simulink model "sistema_completo"  (R2019a)
settings: Solver=VariableStepAuto  StartTime=0.0  StopTime=120  RelTol=1e-3
InitFcn:
  | parametros
values from neighbouring files (symbols this model uses):
  a_h_max = 0.75    [parametros.m]
  a_t_max = 0.8    [parametros.m]
  b_cx = 1.0e6    (= 1000000)    [parametros.m]
  b_cy = 1.0e7    (= 10000000)    [parametros.m]
  b_h_eq = 2 * ( b_hd + i_h^2*b_hm ) / (r_hd^2)    (= 31004.4444444)    [parametros.m]
  b_hb = 1.0e8    (= 100000000)    [parametros.m]
  b_hEb = 2.2e9    (= 2200000000)    [parametros.m]
  b_t = 90.0    (= 90)    [parametros.m]
  b_t_eq = Simulink.Parameter(b_t_eq)    [parametros.m]
  b_tb = 5.0e6    (= 5000000)    [parametros.m]
  b_td_eq = ( b_td + i_t^2*b_tm ) / (r_td^2)    (= 21607.2)    [parametros.m]
  b_tw = 3.0e3    (= 3000)    [parametros.m]
  b_wu = 150    [parametros.m]
  clearance_min = 2    [parametros.m]
  g = Simulink.Parameter(9.80665)    [parametros.m]
  H_c = Simulink.Parameter(2.59)    [parametros.m]
  i_h = 22.0    (= 22)    [parametros.m]
  i_t = 30.0    (= 30)    [parametros.m]
  K_cy = 1.8e9    (= 1800000000)    [parametros.m]
  K_d_h = 2*m_h_eq*xi_hc*w_hc + m_h_eq*p3_hc - b_h_eq    (= 221460.31746)    [parametros.m]
  K_d_t = 2*m_t_eq*xi_tc*w_tc + m_t_eq*p3_tc - b_t_eq.Value    [parametros.m]
  K_i_h = m_h_eq*p3_hc*w_hc^2    (= 25598.9338431)    [parametros.m]
  K_i_t = m_t_eq*p3_tc*w_tc^2    [parametros.m]
  k_p3_th = 3    [parametros.m]
  K_p_h = m_h_eq*w_hc^2 + 2*m_h_eq*xi_hc*w_hc*p3_hc    (= 112940.617295)    [parametros.m]
  K_p_t = m_t_eq*w_tc^2 + 2*m_t_eq*xi_tc*w_tc*p3_tc    [parametros.m]
  k_th = 1    [parametros.m]
  K_tw = 4.8e5    (= 480000)    [parametros.m]
  k_w_c_th = 0.7    [parametros.m]
  k_wu = 2.36e8    (= 236000000)    [parametros.m]
  l_h0 = Y_t0 - y_h0    [parametros.m]
  L_h0 = 110    [parametros.m]
  l_h_man_thresh = 1.0    (= 1)    [parametros.m]
  l_h_tol = 1.0    (= 1)    [parametros.m]
  M_c_max = 50000    [parametros.m]
  M_c_min = 2000    [parametros.m]
  m_h_eq = 2 * ( J_hd_hEb + i_h^2*J_hm_hb ) / (r_hd^2)    (= 65137.7777778)    [parametros.m]
  M_s = 15000    [parametros.m]
  M_t = Simulink.Parameter(30000)    [parametros.m]
  m_td_eq = ( J_td + i_t^2*J_tm_tb ) / (r_td^2)    (= 30000)    [parametros.m]
  N_slots = Simulink.Parameter(floor((x_t_max_oper.Value - x_t_min_oper.Value) / W_c.Value))    [parametros.m]
  overload = false    [parametros.m]
  P_h_nom = 956150    [parametros.m]
  r_hd = 0.75    [parametros.m]
  r_td = 0.50    (= 0.5)    [parametros.m]
  random_obstacles = false    [parametros.m]
  T_hb_max = 5.0e4    (= 50000)    [parametros.m]
  T_hEb_max = 1.1e6    (= 1100000)    [parametros.m]
  T_hm_MAX = 2.0e4    (= 20000)    [parametros.m]
  T_s1 = 20/1000    (= 0.02)    [parametros.m]
  T_s2 = 1/1000    (= 0.001)    [parametros.m]
  T_tb_max = 5.0e3    (= 5000)    [parametros.m]
  T_tm_max = 4.0e3    (= 4000)    [parametros.m]
  tau_hm = 1.0    (= 1)    [parametros.m]
  tau_tm = 1.0    (= 1)    [parametros.m]
  v_h_max = 3.0    (= 3)    [parametros.m]
  v_h_nom = 1.5    [parametros.m]
  v_t_max = 4.0    (= 4)    [parametros.m]
  W_c = Simulink.Parameter(2.44)    [parametros.m]
  w_hm_rated = 2 * (i_h / r_hd) * v_h_nom    (= 88)    [parametros.m]
  x_l0 = x_t0    [parametros.m]
  x_t0 = W_c.Value / 2    [parametros.m]
  x_t_man_thresh = 1.0    (= 1)    [parametros.m]
  x_t_max_emer = x_t_max_oper.Value + 1.0    [parametros.m]
  x_t_max_oper = Simulink.Parameter(50.0)    [parametros.m]
  x_t_min_emer = x_t_min_oper.Value - 1.0    [parametros.m]
  x_t_min_oper = Simulink.Parameter(-30.0)    [parametros.m]
  x_td0 = x_t0    [parametros.m]
  xi_c_th = 0.7    [parametros.m]
  y_c0_0 = Simulink.Parameter(y_c0_ship)    [parametros.m]
  y_c0_quay = 0    [parametros.m]
  y_c0_ship = -20    [parametros.m]
  y_h_max_emer = y_h_max_oper.Value + 1.0    [parametros.m]
  y_h_max_oper = Simulink.Parameter(40.0)    [parametros.m]
  y_h_min_emer = y_h_min_oper.Value - 1.0    [parametros.m]
  y_h_min_oper = Simulink.Parameter(-20.0)    [parametros.m]
  y_l0 = y_h0    [parametros.m]
  Y_t0 = 45.0    (= 45)    [parametros.m]
undefined symbols (not defined in the file or in its folder): DiscIntNeverNeededParam, F_hw, hoist, l_h, l_h_dot, sigbuilder_block, theta_l, theta_l_dot, TLK, translation, x_t_dot
libraries: simulink x10, vrlib x1
(part 1 of 2)
settings Model: EnablePacing=on  Creator=Facundo  LastModifiedBy=Facundo

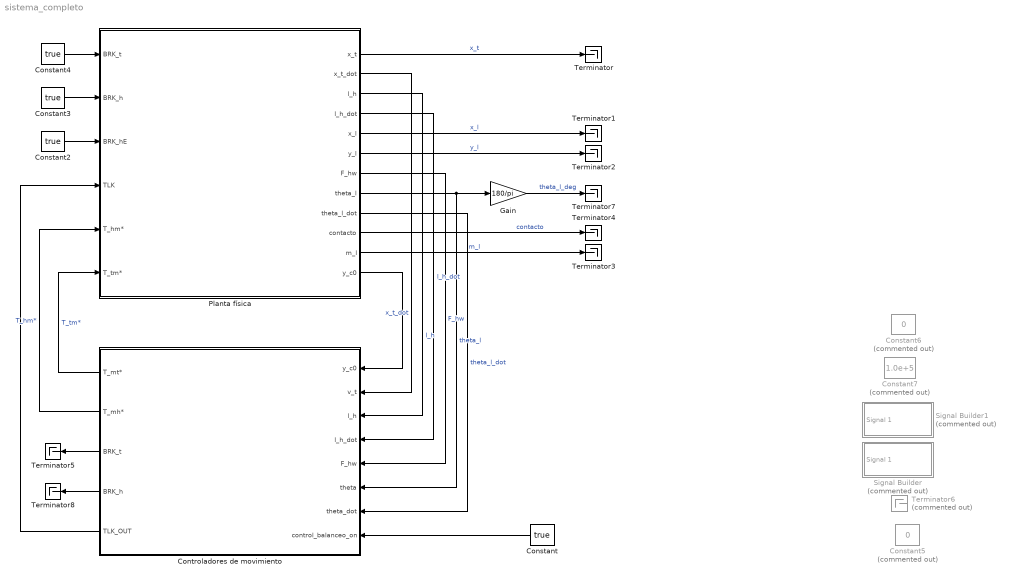
== system sistema_completo ==
  Constant{,2..4} (4 alike) : Constant  Value=true  OutDataTypeStr=boolean
  Constant5 : Constant  Commented=on  Value=0  OutDataTypeStr=boolean
  Constant6 : Constant  Commented=on  Value=0  OutDataTypeStr=double
  Constant7 : Constant  Commented=on  Value=1.0e+5  OutDataTypeStr=double
  Controladores de movimiento : Subsystem
  Gain : Gain  Gain=180/pi
  Planta física : Subsystem
  Signal Builder : Subsystem  Tag=STV Subsys  Commented=on  LoadFcn=sigbuilder_block('load');  StartFcn=sigbuilder_block('start');  StopFcn=sigbuilder_block('stop');  ClipboardFcn=sigbuilder_block('clipboard');  mask(Sigbuilder block){tuvar=[0:10]}
      mask help: Simulink:masks:SigbuilderBlock_MD
      mask init:
      | if ~strcmp(get_param(bdroot(gcbh),'SimulationStatus'),'stopped') tuvar = sigbuilder_block('maskInit'); end
      settings: CopyFcn=sigbuilder_block('copy');  DeleteFcn=sigbuilder_block('delete');  ModelCloseFcn=sigbuilder_block('modelClose');  PreSaveFcn=sigbuilder_block('preSave');  PauseFcn=sigbuilder_block('pause');  ContinueFcn=sigbuilder_block('continue');  NameChangeFcn=sigbuilder_block('namechange');  OpenFcn=sigbuilder_block('open',[5.14286 5.14286 812.571 450.429 ]);  CloseFcn=sigbuilder_block('close');
      mask Display: plot(0, 0, 100, 100,[2, 2, 32, 32, 2], [68, 8, 8, 68, 68],[32, 2], [38, 38], [32, 19, 2],[53, 60, 44], [32, 17, 17, 2],[16, 16, 31, 31]);txt = getActiveGroup(gcbh);text(2, 100, txt,'verticalAlignment', 'top');
  Signal Builder1 : Subsystem  Tag=STV Subsys  Commented=on  LoadFcn=sigbuilder_block('load');  StartFcn=sigbuilder_block('start');  StopFcn=sigbuilder_block('stop');  ClipboardFcn=sigbuilder_block('clipboard');  mask(Sigbuilder block){tuvar=[0:10]}
      mask help: Simulink:masks:SigbuilderBlock_MD
      mask init:
      | if ~strcmp(get_param(bdroot(gcbh),'SimulationStatus'),'stopped') tuvar = sigbuilder_block('maskInit'); end
      settings: CopyFcn=sigbuilder_block('copy');  DeleteFcn=sigbuilder_block('delete');  ModelCloseFcn=sigbuilder_block('modelClose');  PreSaveFcn=sigbuilder_block('preSave');  PauseFcn=sigbuilder_block('pause');  ContinueFcn=sigbuilder_block('continue');  NameChangeFcn=sigbuilder_block('namechange');  OpenFcn=sigbuilder_block('open',[-1152 -103.714 1152 564.429 ]);  CloseFcn=sigbuilder_block('close');
      mask Display: plot(0, 0, 100, 100,[2, 2, 32, 32, 2], [68, 8, 8, 68, 68],[32, 2], [38, 38], [32, 19, 2],[53, 60, 44], [32, 17, 17, 2],[16, 16, 31, 31]);txt = getActiveGroup(gcbh);text(2, 100, txt,'verticalAlignment', 'top');
  Terminator{,1..5,7..8} (8 alike) : Terminator
  Terminator6 : Terminator  Commented=on
  wires:
  Constant/1 -> Controladores de movimiento/8(control_balanceo_on)
  Controladores de movimiento/1(T_mt*) -> Planta física/6(T_tm*)  "T_tm*"
  Controladores de movimiento/2(T_mh*) -> Planta física/5(T_hm*)  "T_hm*"
  Planta física/2(x_t_dot) -> Controladores de movimiento/2(v_t)  "x_t_dot"
  Planta física/4(l_h_dot) -> Controladores de movimiento/4(l_h_dot)  "l_h_dot"
  Planta física/8(theta_l) -> Controladores de movimiento/6(theta), Gain/1  "theta_l"
  Planta física/9(theta_l_dot) -> Controladores de movimiento/7(theta_dot)  "theta_l_dot"
  Planta física/3(l_h) -> Controladores de movimiento/3(l_h)  "l_h"
  Planta física/1(x_t) -> Terminator/1  "x_t"
  Controladores de movimiento/5(TLK_OUT) -> Planta física/4(TLK)
  Constant2/1 -> Planta física/3(BRK_hE)
  Constant3/1 -> Planta física/2(BRK_h)
  Constant4/1 -> Planta física/1(BRK_t)
  Planta física/5(x_l) -> Terminator1/1  "x_l"
  Planta física/6(y_l) -> Terminator2/1  "y_l"
  Planta física/7(F_hw) -> Controladores de movimiento/5(F_hw)  "F_hw"
  Planta física/10(contacto) -> Terminator4/1  "contacto"
  Gain/1 -> Terminator7/1  "theta_l_deg"
  Planta física/11(m_l) -> Terminator3/1  "m_l"
  Controladores de movimiento/3(BRK_t) -> Terminator5/1
  Controladores de movimiento/4(BRK_h) -> Terminator8/1
  Planta física/12(y_c0) -> Controladores de movimiento/1(y_c0)

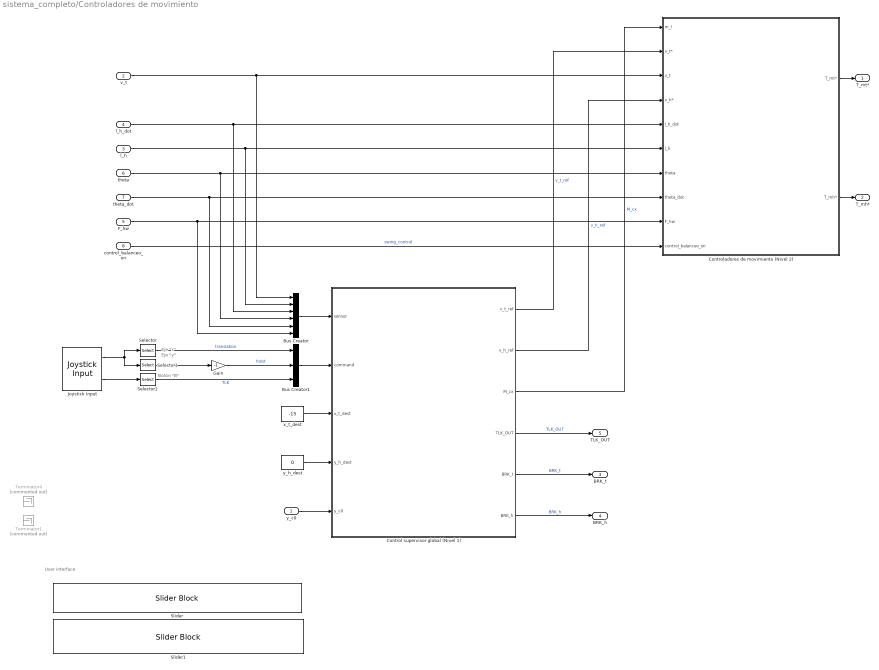
== system sistema_completo/Controladores de movimiento ==
  note: User interface
  note: Botón "B"
  note: Eje "y"
  note: Eje "x"
  y_c0 : Inport  OutDataTypeStr=boolean  LockScale=on
  v_t : Inport  Port=2
  l_h : Inport  Port=3
  l_h_dot : Inport  Port=4
  F_hw : Inport  Port=5
  theta : Inport  Port=6
  theta_dot : Inport  Port=7
  control_balanceo_on : Inport  Port=8  OutDataTypeStr=boolean  LockScale=on
  Bus Creator : BusCreator  Inputs=x_t_dot,l_h,l_h_dot,theta_l,theta_l_dot,F_hw  OutDataTypeStr=Bus: sensor_bus
  Bus Creator1 : BusCreator  Inputs=translation,hoist,TLK  OutDataTypeStr=Bus: command_bus
  Control supervisor global (Nivel 1) : Stateflow chart  BlockKeywords=__PRM__SERIALIZED__DATA__:Stateflow Chart,Stateflow Diagram  TreatAsAtomicUnit=on  SystemSampleTime=T_s1
  Controladores de movimiento (Nivel 2) : Subsystem
  Gain : Gain  Gain=-1
  Joystick Input : vrlib/Joystick Input  joyid=1  adjustports=off  forcefeed=off
      settings: SourceProductName=Simulink
  Selector : Selector  IndexOptions=Index vector (dialog)  Indices=[1]  OutputSizes=1
  Selector1 : Selector  IndexOptions=Index vector (dialog)  Indices=[2]  OutputSizes=1
  Selector2 : Selector  IndexOptions=Index vector (dialog)  Indices=[1]  OutputSizes=1
  Slider : SliderBlock  ScaleMin=-30  ScaleMax=50  TickInterval=5
  Slider1 : SliderBlock  ScaleMin=-20  ScaleMax=40  TickInterval=5
  Terminator1 : Terminator  Commented=on
  Terminator4 : Terminator  Commented=on
  x_t_dest : Constant  Value=-15  OutDataTypeStr=int32
  y_h_dest : Constant  Value=0  OutDataTypeStr=int32
  T_mt* : Outport
  T_mh* : Outport  Port=2
  BRK_t : Outport  Port=3
  BRK_h : Outport  Port=4
  TLK_OUT : Outport  Port=5  OutDataTypeStr=boolean
  wires:
  F_hw/1 -> Bus Creator/6, Controladores de movimiento (Nivel 2)/9(F_hw)
  Controladores de movimiento (Nivel 2)/2(T_mh*) -> T_mh*/1
  Controladores de movimiento (Nivel 2)/1(T_mt*) -> T_mt*/1
  theta/1 -> Bus Creator/4, Controladores de movimiento (Nivel 2)/7(theta)
  control_balanceo_on/1 -> Controladores de movimiento (Nivel 2)/10(control_balanceo_on)  "swing_control"
  theta_dot/1 -> Bus Creator/5, Controladores de movimiento (Nivel 2)/8(theta_dot)
  l_h_dot/1 -> Bus Creator/3, Controladores de movimiento (Nivel 2)/5(l_h_dot)
  v_t/1 -> Bus Creator/1, Controladores de movimiento (Nivel 2)/3(v_t)
  Bus Creator/1 -> Control supervisor global (Nivel 1)/1(sensor)
  l_h/1 -> Controladores de movimiento (Nivel 2)/6(l_h), Bus Creator/2
  Selector/1 -> Bus Creator1/1  "translation"
  Joystick Input/1 -> Selector/1, Selector1/1
  Bus Creator1/1 -> Control supervisor global (Nivel 1)/2(command)
  Control supervisor global (Nivel 1)/1(v_t_ref) -> Controladores de movimiento (Nivel 2)/2(v_t*)  "v_t_ref"
  Control supervisor global (Nivel 1)/2(v_h_ref) -> Controladores de movimiento (Nivel 2)/4(v_h*)  "v_h_ref"
  Control supervisor global (Nivel 1)/5(BRK_t) -> BRK_t/1  "BRK_t"
  Control supervisor global (Nivel 1)/6(BRK_h) -> BRK_h/1  "BRK_h"
  Control supervisor global (Nivel 1)/4(TLK_OUT) -> TLK_OUT/1  "TLK_OUT"
  Control supervisor global (Nivel 1)/3(M_cx) -> Controladores de movimiento (Nivel 2)/1(m_l)  "M_cx"
  Joystick Input/2 -> Selector2/1
  Selector1/1 -> Gain/1
  Selector2/1 -> Bus Creator1/3  "TLK"
  Gain/1 -> Bus Creator1/2  "hoist"
  x_t_dest/1 -> Control supervisor global (Nivel 1)/3(x_t_dest)
  y_h_dest/1 -> Control supervisor global (Nivel 1)/4(y_h_dest)
  y_c0/1 -> Control supervisor global (Nivel 1)/5(y_c0)

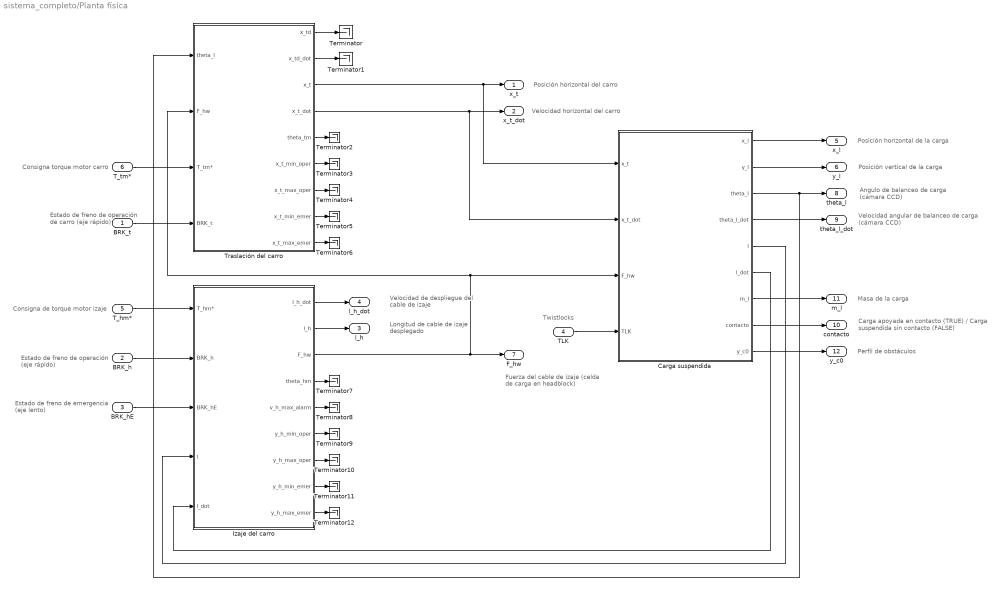
== system sistema_completo/Planta física ==
  note: Consigna de torque motor izaje
  note: Posición horizontal del carro
  note: Velocidad de despliegue
      | del cable de izaje
  note: Longitud de cable
      | de izaje desplegado
  note: Posición horizontal de la carga
  note: Fuerza del cable de izaje
      | (celda de carga en headblock)
  note: Estado de freno de emergencia
      | (eje lento)
  note: Twistlocks
  note: Estado de freno de operación
      | (eje rápido)
  note: Ángulo de balanceo de carga
      | (cámara CCD)
  note: Consigna torque motor carro
  note: Estado de freno de
      | operación de carro
      | (eje rápido)
  note: Posición vertical de la carga
  note: Velocidad horizontal del carro
  note: Velocidad angular de balanceo de carga
      | (cámara CCD)
  note: Masa de la carga
  note: Carga apoyada en contacto (TRUE) /
      | Carga suspendida sin contacto (FALSE)
  note: Perfil de obstáculos
  BRK_t : Inport
  BRK_h : Inport  Port=2
  BRK_hE : Inport  Port=3
  TLK : Inport  Port=4  OutDataTypeStr=boolean  PortDimensions=1  SampleTime=0
  T_hm* : Inport  Port=5
  T_tm* : Inport  Port=6
  Carga suspendida : Subsystem
  Izaje del carro : Subsystem
  Terminator{,1..12} (13 alike) : Terminator
  Traslación del carro : Subsystem
  x_t : Outport
  x_t_dot : Outport  Port=2
  l_h : Outport  Port=3
  l_h_dot : Outport  Port=4
  x_l : Outport  Port=5
  y_l : Outport  Port=6
  F_hw : Outport  Port=7
  theta_l : Outport  Port=8
  theta_l_dot : Outport  Port=9
  contacto : Outport  Port=10
  m_l : Outport  Port=11
  y_c0 : Outport  Port=12
  wires:
  BRK_hE/1 -> Izaje del carro/3(BRK_hE)
  BRK_h/1 -> Izaje del carro/2(BRK_h)
  Traslación del carro/3(x_t) -> Carga suspendida/1(x_t), x_t/1
  BRK_t/1 -> Traslación del carro/4(BRK_t)
  Traslación del carro/1(x_td) -> Terminator/1
  Izaje del carro/1(l_h_dot) -> l_h_dot/1
  Izaje del carro/3(F_hw) -> F_hw/1, Traslación del carro/2(F_hw), Carga suspendida/3(F_hw)
  Carga suspendida/6(l_dot) -> Izaje del carro/5(l_dot)
  Carga suspendida/5(l) -> Izaje del carro/4(l)
  TLK/1 -> Carga suspendida/4(TLK)
  Carga suspendida/3(theta_l) -> Traslación del carro/1(theta_l), theta_l/1
  T_hm*/1 -> Izaje del carro/1(T_hm*)
  Carga suspendida/1(x_l) -> x_l/1
  Izaje del carro/2(l_h) -> l_h/1
  Carga suspendida/2(y_l) -> y_l/1
  Traslación del carro/4(x_t_dot) -> Carga suspendida/2(x_t_dot), x_t_dot/1
  Traslación del carro/2(x_td_dot) -> Terminator1/1
  T_tm*/1 -> Traslación del carro/3(T_tm*)
  Traslación del carro/5(theta_tm) -> Terminator2/1
  Traslación del carro/6(x_t_min_oper) -> Terminator3/1
  Traslación del carro/7(x_t_max_oper) -> Terminator4/1
  Traslación del carro/8(x_t_min_emer) -> Terminator5/1
  Traslación del carro/9(x_t_max_emer) -> Terminator6/1
  Izaje del carro/4(theta_hm) -> Terminator7/1
  Izaje del carro/5(v_h_max_alarm) -> Terminator8/1
  Izaje del carro/6(y_h_min_oper) -> Terminator9/1
  Izaje del carro/7(y_h_max_oper) -> Terminator10/1
  Izaje del carro/8(y_h_min_emer) -> Terminator11/1
  Izaje del carro/9(y_h_max_emer) -> Terminator12/1
  Carga suspendida/4(theta_l_dot) -> theta_l_dot/1
  Carga suspendida/8(contacto) -> contacto/1
  Carga suspendida/7(m_l) -> m_l/1
  Carga suspendida/9(y_c0) -> y_c0/1

== system sistema_completo/Signal Builder ==
  Demux : Demux  Tag=STV Demux  Outputs=1
  FromWs : FromWorkspace  Tag=STV FromWs  VariableName=tuvar  SampleTime=0
      SigBuilderData=|
      | common.afterFinalStr = 'Extrapolate'
      | common.sampleTime = 0
      | dataSet.timeRange = [0 60]
      | dataSet.name = 'Group 1'
      | sbobj.Groups.Name = 'Group 1'
      | sbobj.Groups.Signals.Name = 'Signal 1'
      | sbobj.Groups.Signals.XData = [0 5 15 35 45 60]
      | sbobj.Groups.Signals.YData = [0 0 1 1 0 0]
      | sbobj.Groups.TimeRange = [0 60]
  Signal 1 : Outport  Tag=STV Outport
  wires:
  FromWs/1 -> Demux/1
  Demux/1 -> Signal 1/1

== system sistema_completo/Signal Builder1 ==
  Demux : Demux  Tag=STV Demux  Outputs=1
  FromWs : FromWorkspace  Tag=STV FromWs  VariableName=tuvar  SampleTime=0
      SigBuilderData=|
      | common.afterFinalStr = 'Extrapolate'
      | common.sampleTime = 0
      | dataSet.timeRange = [0 60]
      | dataSet.name = 'Group 1'
      | sbobj.Groups.Name = 'Group 1'
      | sbobj.Groups.Signals.Name = 'Signal 1'
      | sbobj.Groups.Signals.XData = [0 10 20 30 40 60]
      | sbobj.Groups.Signals.YData = [0 0 1 1 0 0]
      | sbobj.Groups.TimeRange = [0 60]
  Signal 1 : Outport  Tag=STV Outport
  wires:
  Demux/1 -> Signal 1/1
  FromWs/1 -> Demux/1

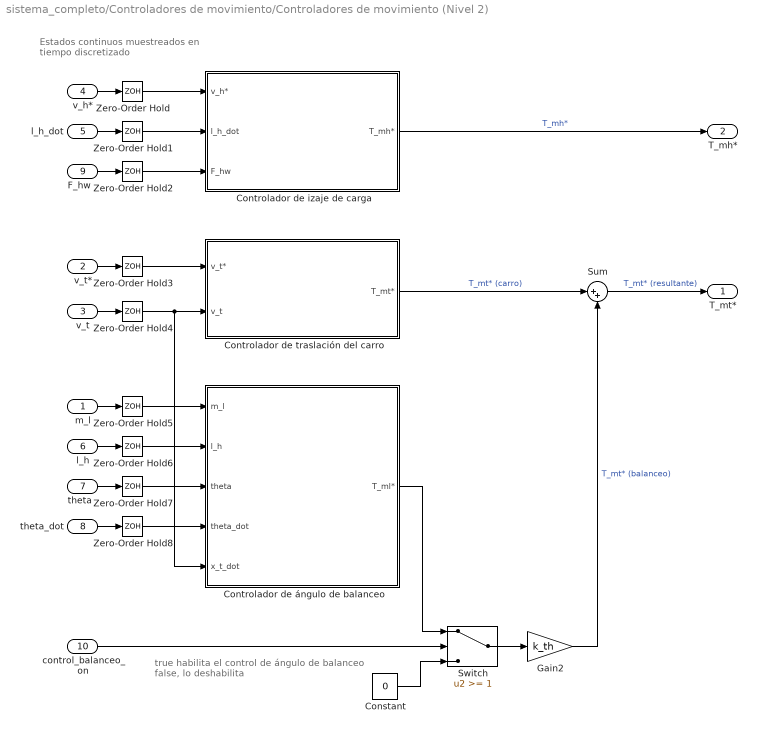
== system sistema_completo/Controladores de movimiento/Controladores de movimiento (Nivel 2) ==
  note: true habilita el control de ángulo de balanceo
      | false, lo deshabilita
  note: Estados continuos muestreados
      | en tiempo discretizado
  m_l : Inport
  v_t* : Inport  Port=2
  v_t : Inport  Port=3
  v_h* : Inport  Port=4
  l_h_dot : Inport  Port=5
  l_h : Inport  Port=6
  theta : Inport  Port=7
  theta_dot : Inport  Port=8
  F_hw : Inport  Port=9
  control_balanceo_on : Inport  Port=10  OutDataTypeStr=boolean  LockScale=on
  Constant : Constant  Value=0
  Controlador de izaje de carga : Subsystem
  Controlador de traslación del carro : Subsystem
  Controlador de ángulo de balanceo : Subsystem
  Gain2 : Gain  Gain=k_th
  Sum : Sum  Inputs=|++
  Switch : Switch  Threshold=1
  Zero-Order Hold{,1..8} (9 alike) : ZeroOrderHold  SampleTime=T_s2
  T_mt* : Outport
  T_mh* : Outport  Port=2
  wires:
  Zero-Order Hold8/1 -> Controlador de ángulo de balanceo/4(theta_dot)
  l_h_dot/1 -> Zero-Order Hold1/1
  Zero-Order Hold5/1 -> Controlador de ángulo de balanceo/1(m_l)
  Zero-Order Hold4/1 -> Controlador de ángulo de balanceo/5(x_t_dot), Controlador de traslación del carro/2(v_t)
  v_t*/1 -> Zero-Order Hold3/1
  theta/1 -> Zero-Order Hold7/1
  Constant/1 -> Switch/3
  Zero-Order Hold3/1 -> Controlador de traslación del carro/1(v_t*)
  v_h*/1 -> Zero-Order Hold/1
  v_t/1 -> Zero-Order Hold4/1
  Zero-Order Hold6/1 -> Controlador de ángulo de balanceo/2(l_h)
  Zero-Order Hold7/1 -> Controlador de ángulo de balanceo/3(theta)
  theta_dot/1 -> Zero-Order Hold8/1
  Sum/1 -> T_mt*/1  "T_mt* (resultante)"
  Zero-Order Hold1/1 -> Controlador de izaje de carga/2(l_h_dot)
  Controlador de izaje de carga/1(T_mh*) -> T_mh*/1  "T_mh*"
  Controlador de traslación del carro/1(T_mt*) -> Sum/1  "T_mt* (carro)"
  m_l/1 -> Zero-Order Hold5/1
  Switch/1 -> Gain2/1
  l_h/1 -> Zero-Order Hold6/1
  Controlador de ángulo de balanceo/1(T_ml*) -> Switch/1
  F_hw/1 -> Zero-Order Hold2/1
  Gain2/1 -> Sum/2  "T_mt* (balanceo)"
  Zero-Order Hold/1 -> Controlador de izaje de carga/1(v_h*)
  Zero-Order Hold2/1 -> Controlador de izaje de carga/3(F_hw)
  control_balanceo_on/1 -> Switch/2

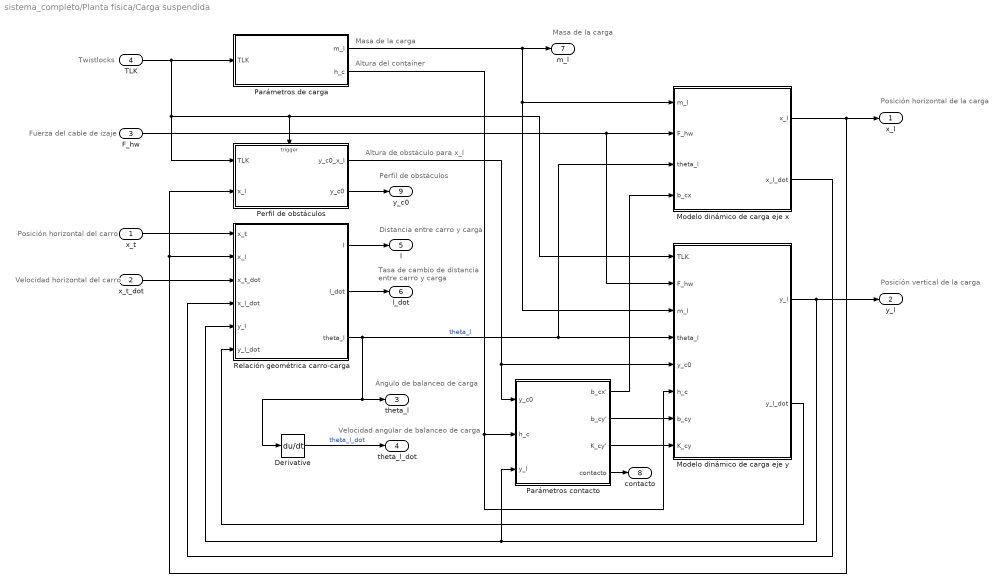
== system sistema_completo/Planta física/Carga suspendida ==
  note: Altura de obstáculo para x_l
  note: Masa de la carga
  note: Twistlocks
  note: Altura del container
  note: Posición horizontal del carro
  note: Posición vertical de la carga
  note: Velocidad horizontal del carro
  note: Distancia entre carro y carga
  note: Fuerza del cable de izaje
  note: Ángulo de balanceo de carga
  note: Tasa de cambio de distancia
      | entre carro y carga
  note: Masa de la carga
  note: Posición horizontal de la carga
  note: Velocidad angular de balanceo de carga
  note: Perfil de obstáculos
  x_t : Inport  OutDataTypeStr=double  PortDimensions=1  SampleTime=0
  x_t_dot : Inport  Port=2  OutDataTypeStr=double  PortDimensions=1  SampleTime=0
  F_hw : Inport  Port=3  OutDataTypeStr=double  PortDimensions=1  SampleTime=0
  TLK : Inport  Port=4  OutDataTypeStr=boolean  PortDimensions=1  SampleTime=0
  Derivative : Derivative
  Modelo dinámico de carga eje x : Subsystem
  Modelo dinámico de carga eje y : Subsystem
  Parámetros contacto : Subsystem
  Parámetros de carga : Subsystem
  Perfil de obstáculos : Subsystem
  Relación geométrica carro-carga : Subsystem
  x_l : Outport  OutDataTypeStr=double  PortDimensions=1  SampleTime=0
  y_l : Outport  Port=2  OutDataTypeStr=double  PortDimensions=1  SampleTime=0
  theta_l : Outport  Port=3  OutDataTypeStr=double  PortDimensions=1  SampleTime=0
  theta_l_dot : Outport  Port=4  OutDataTypeStr=double  PortDimensions=1  SampleTime=0
  l : Outport  Port=5  OutDataTypeStr=double  PortDimensions=1  SampleTime=0
  l_dot : Outport  Port=6  OutDataTypeStr=double  PortDimensions=1  SampleTime=0
  m_l : Outport  Port=7  OutDataTypeStr=double  PortDimensions=1  SampleTime=0
  contacto : Outport  Port=8  OutDataTypeStr=boolean  PortDimensions=1  SampleTime=0
  y_c0 : Outport  Port=9  OutDataTypeStr=double  PortDimensions=1  SampleTime=0
  wires:
  Parámetros de carga/1(m_l) -> Modelo dinámico de carga eje y/3(m_l), Modelo dinámico de carga eje x/1(m_l), m_l/1
  F_hw/1 -> Modelo dinámico de carga eje y/2(F_hw), Modelo dinámico de carga eje x/2(F_hw)
  Relación geométrica carro-carga/2(l_dot) -> l_dot/1
  x_t_dot/1 -> Relación geométrica carro-carga/3(x_t_dot)
  Modelo dinámico de carga eje y/1(y_l) -> Parámetros contacto/3(y_l), Relación geométrica carro-carga/5(y_l), y_l/1
  Modelo dinámico de carga eje x/2(x_l_dot) -> Relación geométrica carro-carga/4(x_l_dot)
  Modelo dinámico de carga eje y/2(y_l_dot) -> Relación geométrica carro-carga/6(y_l_dot)
  x_t/1 -> Relación geométrica carro-carga/1(x_t)
  Modelo dinámico de carga eje x/1(x_l) -> x_l/1, Perfil de obstáculos/2(x_l), Relación geométrica carro-carga/2(x_l)
  Relación geométrica carro-carga/3(theta_l) -> Derivative/1, theta_l/1, Modelo dinámico de carga eje x/3(theta_l), Modelo dinámico de carga eje y/4(theta_l)  "theta_l"
  Parámetros contacto/1(b_cx') -> Modelo dinámico de carga eje x/4(b_cx)
  Parámetros contacto/2(b_cy') -> Modelo dinámico de carga eje y/7(b_cy)
  Parámetros contacto/3(K_cy') -> Modelo dinámico de carga eje y/8(K_cy)
  Relación geométrica carro-carga/1(l) -> l/1
  Parámetros contacto/4(contacto) -> contacto/1
  Parámetros de carga/2(h_c) -> Parámetros contacto/2(h_c), Modelo dinámico de carga eje y/6(h_c)
  Perfil de obstáculos/1(y_c0_x_l) -> Parámetros contacto/1(y_c0), Modelo dinámico de carga eje y/5(y_c0)
  TLK/1 -> Perfil de obstáculos/1(TLK), Perfil de obstáculos/Trigger, Modelo dinámico de carga eje y/1(TLK), Parámetros de carga/1(TLK)
  Derivative/1 -> theta_l_dot/1  "theta_l_dot"
  Perfil de obstáculos/2(y_c0) -> y_c0/1

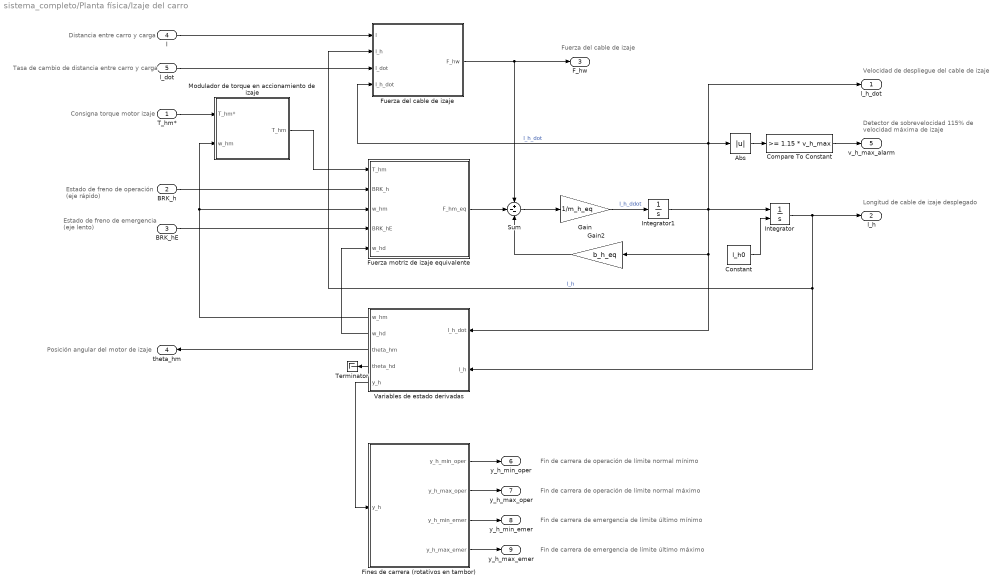
== system sistema_completo/Planta física/Izaje del carro ==
  note: Detector de sobrevelocidad
      | 115% de velocidad máxima de izaje
  note: Posición angular del motor de izaje
  note: Longitud de cable de izaje desplegado
  note: Velocidad de despliegue del cable de izaje
  note: Consigna torque motor izaje
  note: Estado de freno de emergencia
      | (eje lento)
  note: Tasa de cambio de distancia entre carro y carga
  note: Estado de freno de operación
      | (eje rápido)
  note: Distancia entre carro y carga
  note: Fuerza del cable de izaje
  note: Fin de carrera de operación de límite normal mínimo
  note: Fin de carrera de emergencia de límite último máximo
  note: Fin de carrera de emergencia de límite último mínimo
  note: Fin de carrera de operación de límite normal máximo
  T_hm* : Inport
  BRK_h : Inport  Port=2
  BRK_hE : Inport  Port=3
  l : Inport  Port=4
  l_dot : Inport  Port=5
  Abs : Abs
  Compare To Constant : simulink/Logic and Bit Operations/Compare To Constant  relop=>=  const=1.15 * v_h_max  OutDataTypeStr=boolean
  Constant : Constant  Value=l_h0
  Fines de carrera (rotativos en tambor) : Subsystem
  Fuerza del cable de izaje : Subsystem
  Fuerza motriz de izaje equivalente : Subsystem
  Gain : Gain  Gain=1/m_h_eq
  Gain2 : Gain  Gain=b_h_eq
  Integrator : Integrator  InitialConditionSource=external
  Integrator1 : Integrator
  Modulador de torque en accionamiento de izaje : Subsystem
  Sum : Sum  Inputs=+--
  Terminator : Terminator
  Variables de estado derivadas : Subsystem
  l_h_dot : Outport
  l_h : Outport  Port=2
  F_hw : Outport  Port=3
  theta_hm : Outport  Port=4
  v_h_max_alarm : Outport  Port=5
  y_h_min_oper : Outport  Port=6  OutDataTypeStr=boolean  PortDimensions=1  SampleTime=0
  y_h_max_oper : Outport  Port=7  OutDataTypeStr=boolean  PortDimensions=1  SampleTime=0
  y_h_min_emer : Outport  Port=8  OutDataTypeStr=boolean  PortDimensions=1  SampleTime=0
  y_h_max_emer : Outport  Port=9  OutDataTypeStr=boolean  PortDimensions=1  SampleTime=0
  wires:
  Integrator/1 -> l_h/1, Variables de estado derivadas/2(l_h), Fuerza del cable de izaje/2(l_h)  "l_h"
  Integrator1/1 -> l_h_dot/1, Fuerza del cable de izaje/4(l_h_dot), Abs/1, Variables de estado derivadas/1(l_h_dot), Gain2/1, Integrator/1  "l_h_dot"
  l/1 -> Fuerza del cable de izaje/1(l)
  l_dot/1 -> Fuerza del cable de izaje/3(l_dot)
  Fuerza del cable de izaje/1(F_hw) -> F_hw/1, Sum/1
  Gain2/1 -> Sum/3
  Fuerza motriz de izaje equivalente/1(F_hm_eq) -> Sum/2
  Variables de estado derivadas/1(w_hm) -> Fuerza motriz de izaje equivalente/3(w_hm), Modulador de torque en accionamiento de izaje/2(w_hm)
  Sum/1 -> Gain/1
  Variables de estado derivadas/2(w_hd) -> Fuerza motriz de izaje equivalente/5(w_hd)
  BRK_h/1 -> Fuerza motriz de izaje equivalente/2(BRK_h)
  BRK_hE/1 -> Fuerza motriz de izaje equivalente/4(BRK_hE)
  Gain/1 -> Integrator1/1  "l_h_ddot"
  Constant/1 -> Integrator/2
  Variables de estado derivadas/3(theta_hm) -> theta_hm/1
  Abs/1 -> Compare To Constant/1
  Compare To Constant/1 -> v_h_max_alarm/1
  Fines de carrera (rotativos en tambor)/1(y_h_min_oper) -> y_h_min_oper/1
  Fines de carrera (rotativos en tambor)/4(y_h_max_emer) -> y_h_max_emer/1
  Fines de carrera (rotativos en tambor)/3(y_h_min_emer) -> y_h_min_emer/1
  Fines de carrera (rotativos en tambor)/2(y_h_max_oper) -> y_h_max_oper/1
  Variables de estado derivadas/5(y_h) -> Fines de carrera (rotativos en tambor)/1(y_h)
  Variables de estado derivadas/4(theta_hd) -> Terminator/1
  Modulador de torque en accionamiento de izaje/1(T_hm) -> Fuerza motriz de izaje equivalente/1(T_hm)
  T_hm*/1 -> Modulador de torque en accionamiento de izaje/1(T_hm*)

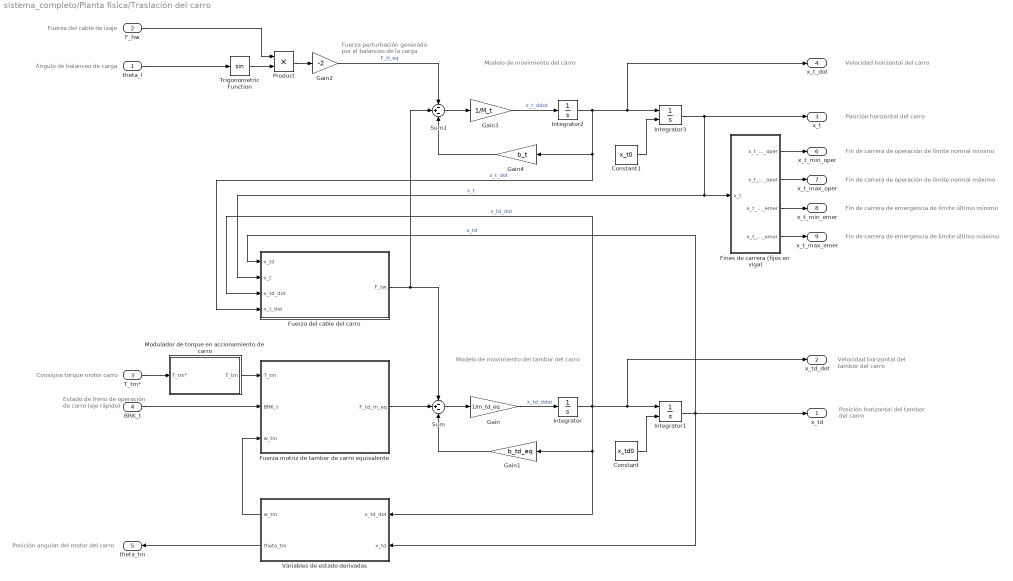
== system sistema_completo/Planta física/Traslación del carro ==
  note: Posición angular del motor del carro
  note: Velocidad horizontal
      | del tambor del carro
  note: Modelo de movimiento del tambor del carro
  note: Modelo de movimiento del carro
  note: Velocidad horizontal del carro
  note: Estado de freno de
      | operación de carro
      | (eje rápido)
  note: Fuerza del cable de izaje
  note: Fuerza perturbación generada
      | por el balanceo de la carga
  note: Posición horizontal del carro
  note: Consigna torque motor carro
  note: Ángulo de balanceo de carga
  note: Posición horizontal
      | del tambor del carro
  note: Fin de carrera de operación de límite normal mínimo
  note: Fin de carrera de operación de límite normal máximo
  note: Fin de carrera de emergencia de límite último mínimo
  note: Fin de carrera de emergencia de límite último máximo
  theta_l : Inport  OutDataTypeStr=double  PortDimensions=1  SampleTime=0
  F_hw : Inport  Port=2  OutDataTypeStr=double  PortDimensions=1  SampleTime=0
  T_tm* : Inport  Port=3
  BRK_t : Inport  Port=4
  Constant : Constant  Value=x_td0
  Constant1 : Constant  Value=x_t0
  Fines de carrera (fijos en viga) : Subsystem
  Fuerza del cable del carro : Subsystem
  Fuerza motriz de tambor de carro equivalente : Subsystem
  Gain : Gain  Gain=1/m_td_eq
  Gain1 : Gain  Gain=b_td_eq
  Gain2 : Gain  Gain=-2
  Gain3 : Gain  Gain=1/M_t
  Gain4 : Gain  Gain=b_t
  Integrator : Integrator
  Integrator1 : Integrator  InitialConditionSource=external
  Integrator2 : Integrator
  Integrator3 : Integrator  InitialConditionSource=external
  Modulador de torque en accionamiento de carro : Subsystem
  Product : Product
  Sum : Sum  Inputs=-+-
  Sum1 : Sum  Inputs=-+-
  Trigonometric Function : Trigonometry
  Variables de estado derivadas : Subsystem
  x_td : Outport  OutDataTypeStr=double  PortDimensions=1  SampleTime=0
  x_td_dot : Outport  Port=2  OutDataTypeStr=double  PortDimensions=1  SampleTime=0
  x_t : Outport  Port=3  OutDataTypeStr=double  PortDimensions=1  SampleTime=0
  x_t_dot : Outport  Port=4  OutDataTypeStr=double  PortDimensions=1  SampleTime=0
  theta_tm : Outport  Port=5  OutDataTypeStr=double  PortDimensions=1  SampleTime=0
  x_t_min_oper : Outport  Port=6  OutDataTypeStr=boolean  PortDimensions=1  SampleTime=0
  x_t_max_oper : Outport  Port=7  OutDataTypeStr=boolean  PortDimensions=1  SampleTime=0
  x_t_min_emer : Outport  Port=8  OutDataTypeStr=boolean  PortDimensions=1  SampleTime=0
  x_t_max_emer : Outport  Port=9  OutDataTypeStr=boolean  PortDimensions=1  SampleTime=0
  wires:
  Integrator1/1 -> Variables de estado derivadas/2(x_td), Fuerza del cable del carro/1(x_td), x_td/1  "x_td"
  Gain3/1 -> Integrator2/1  "x_t_ddot"
  Fuerza del cable del carro/1(F_tw) -> Sum1/2, Sum/1
  Sum/1 -> Gain/1
  Integrator/1 -> Fuerza del cable del carro/3(x_td_dot), Variables de estado derivadas/1(x_td_dot), Gain1/1, x_td_dot/1, Integrator1/1  "x_td_dot"
  F_hw/1 -> Product/1
  Fuerza motriz de tambor de carro equivalente/1(F_td_m_eq) -> Sum/2
  Constant/1 -> Integrator1/2
  Gain1/1 -> Sum/3
  Integrator2/1 -> Fuerza del cable del carro/4(x_t_dot), Gain4/1, x_t_dot/1, Integrator3/1  "x_t_dot"
  Sum1/1 -> Gain3/1
  theta_l/1 -> Trigonometric Function/1
  Gain4/1 -> Sum1/3
  Integrator3/1 -> x_t/1, Fuerza del cable del carro/2(x_t), Fines de carrera (fijos en viga)/1(x_t)  "x_t"
  Gain2/1 -> Sum1/1  "F_tl_eq"
  T_tm*/1 -> Modulador de torque en accionamiento de carro/1(T_tm*)
  BRK_t/1 -> Fuerza motriz de tambor de carro equivalente/2(BRK_t)
  Variables de estado derivadas/1(w_tm) -> Fuerza motriz de tambor de carro equivalente/3(w_tm)
  Constant1/1 -> Integrator3/2
  Trigonometric Function/1 -> Product/2
  Product/1 -> Gain2/1
  Gain/1 -> Integrator/1  "x_td_ddot"
  Variables de estado derivadas/2(theta_tm) -> theta_tm/1
  Fines de carrera (fijos en viga)/1(x_t_min_oper) -> x_t_min_oper/1
  Fines de carrera (fijos en viga)/2(x_t_max_oper) -> x_t_max_oper/1
  Fines de carrera (fijos en viga)/3(x_t_min_emer) -> x_t_min_emer/1
  Fines de carrera (fijos en viga)/4(x_t_max_emer) -> x_t_max_emer/1
  Modulador de torque en accionamiento de carro/1(T_tm) -> Fuerza motriz de tambor de carro equivalente/1(T_tm)

== system sistema_completo/Controladores de movimiento/Controladores de movimiento (Nivel 2)/Controlador de izaje de carga ==
  v_h* : Inport
  l_h_dot : Inport  Port=2
  F_hw : Inport  Port=3
  Discrete-Time Integrator : DiscreteIntegrator  SampleTime=T_s2  ICPrevOutput=DiscIntNeverNeededParam  ICPrevScaledInput=DiscIntNeverNeededParam
  Discrete-Time Integrator1 : DiscreteIntegrator  SampleTime=T_s2  ICPrevOutput=DiscIntNeverNeededParam  ICPrevScaledInput=DiscIntNeverNeededParam
  Gain : Gain  Gain=K_d_h
  Gain1 : Gain  Gain=-1
  Gain2 : Gain  Gain=K_p_h
  Gain3 : Gain  Gain=K_i_h
  Gain5 : Gain  Gain=r_hd/i_h
  Sum : Sum  Inputs=+++
  Sum1 : Sum  Inputs=|+-
  Sum2 : Sum  Inputs=|-+
  T_mh* : Outport
  wires:
  Discrete-Time Integrator1/1 -> Gain3/1
  Gain/1 -> Sum/3  "acción D"
  v_h*/1 -> Gain1/1  "v_h*"
  Discrete-Time Integrator/1 -> Gain2/1, Discrete-Time Integrator1/1
  Gain3/1 -> Sum/1  "acción I"
  Gain2/1 -> Sum/2  "acción P"
  Sum/1 -> Sum2/1  "F_h_eq_total*"
  Sum1/1 -> Discrete-Time Integrator/1, Gain/1  "e_l_h"
  Gain1/1 -> Sum1/1  "l_h_dot*"
  l_h_dot/1 -> Sum1/2  "l_h_dot"
  Gain5/1 -> T_mh*/1  "T_mh*"
  F_hw/1 -> Sum2/2  "F_hw"
  Sum2/1 -> Gain5/1

== system sistema_completo/Controladores de movimiento/Controladores de movimiento (Nivel 2)/Controlador de traslación del carro ==
  v_t* : Inport
  v_t : Inport  Port=2
  Discrete-Time Integrator : DiscreteIntegrator  SampleTime=T_s2  ICPrevOutput=DiscIntNeverNeededParam  ICPrevScaledInput=DiscIntNeverNeededParam
  Discrete-Time Integrator1 : DiscreteIntegrator  SampleTime=T_s2  ICPrevOutput=DiscIntNeverNeededParam  ICPrevScaledInput=DiscIntNeverNeededParam
  Gain : Gain  Gain=K_d_t
  Gain1 : Gain  Gain=r_td/i_t
  Gain2 : Gain  Gain=K_p_t
  Gain3 : Gain  Gain=K_i_t
  Sum : Sum  Inputs=+++
  Sum1 : Sum  Inputs=|+-
  T_mt* : Outport
  wires:
  v_t/1 -> Sum1/2
  Discrete-Time Integrator/1 -> Discrete-Time Integrator1/1, Gain2/1
  Gain2/1 -> Sum/2  "acción P"
  Gain3/1 -> Sum/1  "acción I"
  Sum1/1 -> Discrete-Time Integrator/1, Gain/1  "e_v_t"
  v_t*/1 -> Sum1/1
  Discrete-Time Integrator1/1 -> Gain3/1
  Gain/1 -> Sum/3  "acción D"
  Sum/1 -> Gain1/1  "F_t_eq*"
  Gain1/1 -> T_mt*/1  "T_mt*"

== system sistema_completo/Controladores de movimiento/Controladores de movimiento (Nivel 2)/Controlador de ángulo de balanceo ==
  note: Entrada virtual
      | al subsistema
  note: Nota:
      | e_theta = theta* - theta
      | theta* = 0 (consigna)
      |
      | Entonces
      | e_theta = - theta
      | e_theta_dot = - theta_dot
  note: Variable de ajuste
  note: Salida del
      | subsistema
  note: Entrada real
      | al subsistema
  m_l : Inport
  l_h : Inport  Port=2
  theta : Inport  Port=3
  theta_dot : Inport  Port=4
  x_t_dot : Inport  Port=5
  Des-linearización por retroalimentación : Subsystem
  Discrete-Time Integrator : DiscreteIntegrator  SampleTime=T_s2  ICPrevOutput=DiscIntNeverNeededParam  ICPrevScaledInput=DiscIntNeverNeededParam
  Gain : Gain  Gain=-1
  Gain1 : Gain  Gain=-1
  Gain2 : Gain  Gain=r_td/i_t
  Ganancias programadas : Subsystem
  Product : Product
  Product1 : Product
  Product2 : Product
  Sum : Sum  Inputs=+++
  T_ml* : Outport
  wires:
  Product1/1 -> Sum/2  "acción P"
  Product/1 -> Sum/1  "acción I"
  Discrete-Time Integrator/1 -> Product/2
  Product2/1 -> Sum/3  "acción D"
  Ganancias programadas/1(K_p_th) -> Product/1
  Ganancias programadas/2(K_i_th) -> Product1/1
  Ganancias programadas/3(K_d_th) -> Product2/1
  l_h/1 -> Des-linearización por retroalimentación/6(l_h), Ganancias programadas/1(l_h)
  Gain1/1 -> Product2/2  "e_theta_dot"
  theta/1 -> Gain/1
  theta_dot/1 -> Des-linearización por retroalimentación/4(theta_dot), Gain1/1
  Sum/1 -> Des-linearización por retroalimentación/2(v)  "v(t)"
  x_t_dot/1 -> Des-linearización por retroalimentación/5(x_t_dot)
  Des-linearización por retroalimentación/1(F_t_eq) -> Gain2/1
  Gain2/1 -> T_ml*/1
  m_l/1 -> Des-linearización por retroalimentación/1(m_l)
  Gain/1 -> Discrete-Time Integrator/1, Product1/2, Des-linearización por retroalimentación/3(theta)  "e_theta"

== system sistema_completo/Planta física/Carga suspendida/Modelo dinámico de carga eje x ==
  note: Componente horizontal de
      | fuerza del cable de izaje
  note: Posición horizontal de la carga
  note: Velocidad horizontal de la carga
  note: Fuerza del cable de izaje
  note: Masa de la carga
  note: Fricción por contacto
      | horizontal (arrastre)
  note: Ángulo de balanceo de carga
  m_l : Inport  OutDataTypeStr=double  PortDimensions=1  SampleTime=0
  F_hw : Inport  Port=2  OutDataTypeStr=double  PortDimensions=1  SampleTime=0
  theta_l : Inport  Port=3  OutDataTypeStr=double  PortDimensions=1  SampleTime=0
  b_cx : Inport  Port=4  OutDataTypeStr=double  PortDimensions=1  SampleTime=0
  Constant : Constant  Value=x_l0
  Divide : Product  Inputs=*/
  Gain2 : Gain  Gain=-2
  Integrator : Integrator
  Integrator1 : Integrator  InitialConditionSource=external
  Product : Product
  Product1 : Product
  Sum : Sum  Inputs=|+-
  Trigonometric Function : Trigonometry
  x_l : Outport  OutDataTypeStr=double  PortDimensions=1  SampleTime=0
  x_l_dot : Outport  Port=2  OutDataTypeStr=double  PortDimensions=1  SampleTime=0
  wires:
  F_hw/1 -> Product/1
  Product1/1 -> Sum/2
  theta_l/1 -> Trigonometric Function/1
  b_cx/1 -> Product1/2
  Sum/1 -> Divide/1
  Integrator/1 -> x_l_dot/1, Integrator1/1, Product1/1  "x_l_dot"
  Product/1 -> Gain2/1
  Divide/1 -> Integrator/1  "x_l_ddot"
  Constant/1 -> Integrator1/2
  Integrator1/1 -> x_l/1
  Gain2/1 -> Sum/1
  m_l/1 -> Divide/2
  Trigonometric Function/1 -> Product/2

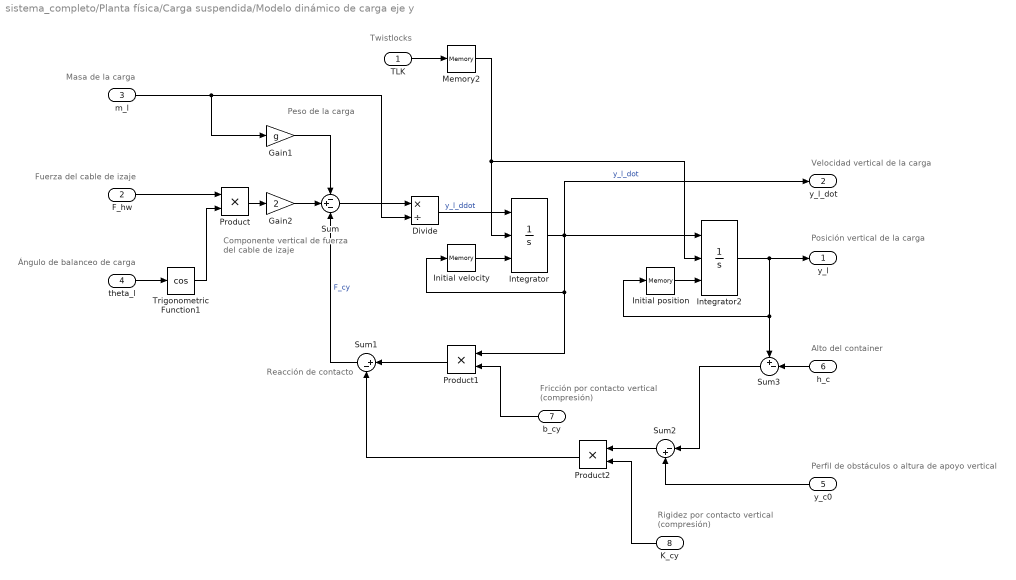
== system sistema_completo/Planta física/Carga suspendida/Modelo dinámico de carga eje y ==
  note: Twistlocks
  note: Reacción de contacto
  note: Peso de la carga
  note: Componente vertical de
      | fuerza del cable de izaje
  note: Posición vertical de la carga
  note: Velocidad vertical de la carga
  note: Fricción por contacto
      | vertical (compresión)
  note: Rigidez por contacto
      | vertical (compresión)
  note: Masa de la carga
  note: Fuerza del cable de izaje
  note: Perfil de obstáculos o altura de apoyo vertical
  note: Alto del container
  note: Ángulo de balanceo de carga
  TLK : Inport  OutDataTypeStr=boolean  PortDimensions=1  SampleTime=0
  F_hw : Inport  Port=2  OutDataTypeStr=double  PortDimensions=1  SampleTime=0
  m_l : Inport  Port=3  OutDataTypeStr=double  PortDimensions=1  SampleTime=0
  theta_l : Inport  Port=4  OutDataTypeStr=double  PortDimensions=1  SampleTime=0
  y_c0 : Inport  Port=5  OutDataTypeStr=double  PortDimensions=1  SampleTime=0
  h_c : Inport  Port=6  OutDataTypeStr=double  PortDimensions=1  SampleTime=0
  b_cy : Inport  Port=7  OutDataTypeStr=double  PortDimensions=1  SampleTime=0
  K_cy : Inport  Port=8  OutDataTypeStr=double  PortDimensions=1  SampleTime=0
  Divide : Product  Inputs=*/
  Gain1 : Gain  Gain=g
  Gain2 : Gain  Gain=2
  Initial position : Memory  InitialCondition=y_l0  InheritSampleTime=on  LinearizeAsDelay=on
  Initial velocity : Memory  InheritSampleTime=on  LinearizeAsDelay=on
  Integrator : Integrator  ExternalReset=either  InitialConditionSource=external
  Integrator2 : Integrator  ExternalReset=either  InitialConditionSource=external
  Memory2 : Memory  InitialCondition=false  InheritSampleTime=on  LinearizeAsDelay=on
  Product : Product
  Product1 : Product
  Product2 : Product
  Sum : Sum  Inputs=-+-
  Sum1 : Sum  Inputs=|+-
  Sum2 : Sum  Inputs=|-+
  Sum3 : Sum  Inputs=+-|
  Trigonometric Function1 : Trigonometry  Operator=cos
  y_l : Outport  OutDataTypeStr=double  PortDimensions=1  SampleTime=0
  y_l_dot : Outport  Port=2  OutDataTypeStr=double  PortDimensions=1  SampleTime=0
  wires:
  F_hw/1 -> Product/1
  theta_l/1 -> Trigonometric Function1/1
  b_cy/1 -> Product1/2
  Integrator/1 -> y_l_dot/1, Integrator2/1, Initial velocity/1, Product1/1  "y_l_dot"
  Divide/1 -> Integrator/1  "y_l_ddot"
  Integrator2/1 -> y_l/1, Sum3/1, Initial position/1
  Product/1 -> Gain2/1
  Product1/1 -> Sum1/1
  Sum1/1 -> Sum/3  "F_cy"
  Gain1/1 -> Sum/1
  y_c0/1 -> Sum2/2
  Sum2/1 -> Product2/1
  K_cy/1 -> Product2/2
  Product2/1 -> Sum1/2
  Gain2/1 -> Sum/2
  Sum/1 -> Divide/1
  m_l/1 -> Gain1/1, Divide/2
  h_c/1 -> Sum3/2
  Sum3/1 -> Sum2/1
  Trigonometric Function1/1 -> Product/2
  Initial velocity/1 -> Integrator/3
  Initial position/1 -> Integrator2/3
  TLK/1 -> Memory2/1
  Memory2/1 -> Integrator2/2, Integrator/2

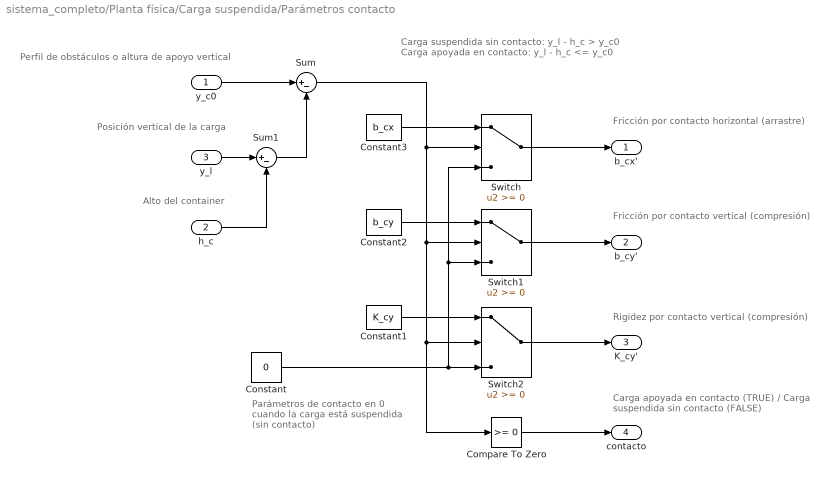
== system sistema_completo/Planta física/Carga suspendida/Parámetros contacto ==
  note: Fricción por contacto horizontal (arrastre)
  note: Fricción por contacto vertical (compresión)
  note: Rigidez por contacto vertical (compresión)
  note: Perfil de obstáculos o altura de apoyo vertical
  note: Posición vertical de la carga
  note: Alto del container
  note: Parámetros de contacto en 0
      | cuando la carga está suspendida
      | (sin contacto)
  note: Carga suspendida sin contacto: y_l - h_c > y_c0
      | Carga apoyada en contacto: y_l - h_c <= y_c0
  note: Carga apoyada en contacto (TRUE) /
      | Carga suspendida sin contacto (FALSE)
  y_c0 : Inport  OutDataTypeStr=double  PortDimensions=1  SampleTime=0
  h_c : Inport  Port=2  OutDataTypeStr=double  PortDimensions=1  SampleTime=0
  y_l : Inport  Port=3  OutDataTypeStr=double  PortDimensions=1  SampleTime=0
  Compare To Zero : simulink/Logic and Bit Operations/Compare To Zero  relop=>=  OutDataTypeStr=boolean
  Constant : Constant  Value=0
  Constant1 : Constant  Value=K_cy
  Constant2 : Constant  Value=b_cy
  Constant3 : Constant  Value=b_cx
  Sum : Sum  Inputs=|+-
  Sum1 : Sum  Inputs=|+-
  Switch : Switch
  Switch1 : Switch
  Switch2 : Switch
  b_cx' : Outport  OutDataTypeStr=double  PortDimensions=1  SampleTime=0
  b_cy' : Outport  Port=2  OutDataTypeStr=double  PortDimensions=1  SampleTime=0
  K_cy' : Outport  Port=3  OutDataTypeStr=double  PortDimensions=1  SampleTime=0
  contacto : Outport  Port=4  OutDataTypeStr=boolean  PortDimensions=1  SampleTime=0
  wires:
  y_c0/1 -> Sum/1
  Constant2/1 -> Switch1/1
  Constant1/1 -> Switch2/1
  Switch/1 -> b_cx'/1
  Sum/1 -> Switch1/2, Compare To Zero/1, Switch2/2, Switch/2
  Switch2/1 -> K_cy'/1
  Switch1/1 -> b_cy'/1
  Constant/1 -> Switch/3, Switch1/3, Switch2/3
  Constant3/1 -> Switch/1
  Sum1/1 -> Sum/2
  y_l/1 -> Sum1/1
  h_c/1 -> Sum1/2
  Compare To Zero/1 -> contacto/1

== system sistema_completo/Planta física/Carga suspendida/Parámetros de carga ==
  note: Twistlocks
  note: Masa de la carga total
  note: Alto del container
      | (afecta altura inferior)
  note: Masa del spreader
  note: Masa del contenedor
      | y carga
  TLK : Inport  OutDataTypeStr=boolean  PortDimensions=1  SampleTime=0
  "Generate random load " : Subsystem  TreatAsAtomicUnit=on
  Sum : Sum  Inputs=++|
  Switch : Switch  Criteria=u2 ~= 0
  Switch1 : Switch  Criteria=u2 ~= 0
  h_c1 : Constant  Value=H_c
  h_c2 : Constant  Value=0
  h_c3 : Constant  Value=M_s
  h_c4 : Constant  Value=0
  m_l : Outport
  h_c : Outport  Port=2
  wires:
  TLK/1 -> "Generate random load "/Trigger, Switch1/2, Switch/2
  Switch/1 -> h_c/1
  Sum/1 -> m_l/1
  Switch1/1 -> Sum/2  "M_cx"
  "Generate random load "/1(M_cx) -> Switch1/1
  h_c3/1 -> Sum/1  "M_s"
  h_c2/1 -> Switch/3
  h_c4/1 -> Switch1/3
  h_c1/1 -> Switch/1

== system sistema_completo/Planta física/Carga suspendida/Perfil de obstáculos ==
  note: Perfil de obstáculos para x_l
  note: Se actualiza el perfil de obstá culos cuando
      | se cierran (TLK ↑) o abren (TLK ↓) los twistlocks
  note: Perfil de obstáculos
  note: Guarda perfil de obstáculos en workspace
      | para posterior análisis (plot_perfil_obstaculos.m)
  TLK : Inport  PortDimensions=1
  x_l : Inport  Port=2  OutDataTypeStr=double  PortDimensions=1
  Trigger : TriggerPort  TriggerType=either  VariantControl=Variant  PortDimensions=1
  MATLAB Function : MATLAB Function  TreatAsAtomicUnit=on
  To Workspace : ToWorkspace  VariableName=y_c0  SaveFormat=Structure With Time  SampleTime=-1
  y_c0_x_l : Outport  OutDataTypeStr=double  PortDimensions=1  InitialOutput=y_c0_0
  y_c0 : Outport  Port=2  OutDataTypeStr=double  PortDimensions=1  InitialOutput=y_c0_0
  wires:
  MATLAB Function/1(y_c0_x_l) -> y_c0_x_l/1
  TLK/1 -> MATLAB Function/2(TLK)
  x_l/1 -> MATLAB Function/1(x_l)
  MATLAB Function/2(y_c0) -> y_c0/1, To Workspace/1

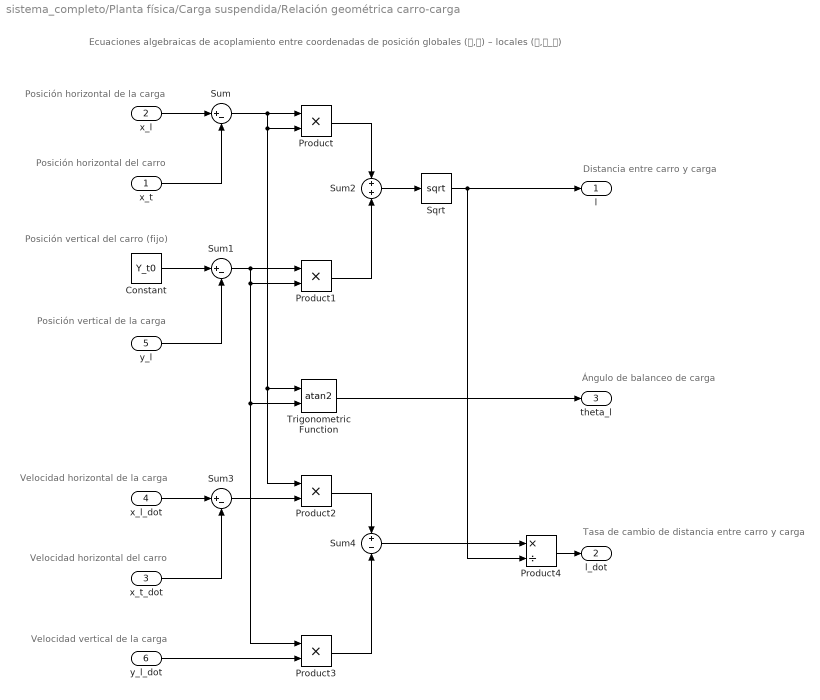
== system sistema_completo/Planta física/Carga suspendida/Relación geométrica carro-carga ==
  note: Ecuaciones algebraicas de acoplamiento entre coordenadas de posición globales (𝑥,𝑦) – locales (𝑙,𝜃_𝑙)
  note: Posición horizontal de la carga
  note: Posición horizontal del carro
  note: Posición vertical del carro (fijo)
  note: Posición vertical de la carga
  note: Distancia entre carro y carga
  note: Tasa de cambio de distancia entre carro y carga
  note: Ángulo de balanceo de carga
  note: Velocidad horizontal de la carga
  note: Velocidad horizontal del carro
  note: Velocidad vertical de la carga
  x_t : Inport
  x_l : Inport  Port=2
  x_t_dot : Inport  Port=3
  x_l_dot : Inport  Port=4
  y_l : Inport  Port=5
  y_l_dot : Inport  Port=6
  Constant : Constant  Value=Y_t0
  Product{,1..3} (4 alike) : Product
  Product4 : Product  Inputs=*/
  Sqrt : Sqrt  SaturateOnIntegerOverflow=on
  Sum : Sum  Inputs=|+-
  Sum1 : Sum  Inputs=|+-
  Sum2 : Sum  Inputs=+|+
  Sum3 : Sum  Inputs=|+-
  Sum4 : Sum  Inputs=+|-
  Trigonometric Function : Trigonometry  Operator=atan2
  l : Outport
  l_dot : Outport  Port=2
  theta_l : Outport  Port=3
  wires:
  x_t/1 -> Sum/2
  x_l/1 -> Sum/1
  Sum/1 -> Product/1, Product2/1, Trigonometric Function/1, Product/2
  Product/1 -> Sum2/1
  y_l/1 -> Sum1/2
  Sum1/1 -> Product1/1, Product3/1, Trigonometric Function/2, Product1/2
  Constant/1 -> Sum1/1
  Product1/1 -> Sum2/2
  Sum2/1 -> Sqrt/1
  Trigonometric Function/1 -> theta_l/1
  x_l_dot/1 -> Sum3/1
  x_t_dot/1 -> Sum3/2
  Sum3/1 -> Product2/2
  y_l_dot/1 -> Product3/2
  Product2/1 -> Sum4/1
  Product3/1 -> Sum4/2
  Sum4/1 -> Product4/1
  Product4/1 -> l_dot/1
  Sqrt/1 -> Product4/2, l/1

== system sistema_completo/Planta física/Izaje del carro/Fines de carrera (rotativos en tambor) ==
  note: Fines de carrera son rotativos sobre tambor (theta_hd). Por simplicidad se usa la variable equivalente lineal (y_h)
  note: Fin de carrera de operación de límite normal mínimo
  note: Fin de carrera de operación de límite normal máximo
  note: Fin de carrera de emergencia de límite último mínimo
  note: Fin de carrera de operación de límite último máximo
  note: Altura de la carga sin balanceo
  y_h : Inport
  Compare To Constant : simulink/Logic and Bit Operations/Compare To Constant  relop=<=  const=y_h_min_oper  OutDataTypeStr=boolean
  Compare To Constant1 : simulink/Logic and Bit Operations/Compare To Constant  relop=>=  const=y_h_max_oper  OutDataTypeStr=boolean
  Compare To Constant2 : simulink/Logic and Bit Operations/Compare To Constant  relop=<=  const=y_h_min_emer  OutDataTypeStr=boolean
  Compare To Constant3 : simulink/Logic and Bit Operations/Compare To Constant  relop=>=  const=y_h_max_emer  OutDataTypeStr=boolean
  y_h_min_oper : Outport  OutDataTypeStr=boolean  PortDimensions=1  SampleTime=0
  y_h_max_oper : Outport  Port=2  OutDataTypeStr=boolean  PortDimensions=1  SampleTime=0
  y_h_min_emer : Outport  Port=3  OutDataTypeStr=boolean  PortDimensions=1  SampleTime=0
  y_h_max_emer : Outport  Port=4  OutDataTypeStr=boolean  PortDimensions=1  SampleTime=0
  wires:
  Compare To Constant2/1 -> y_h_min_emer/1
  Compare To Constant/1 -> y_h_min_oper/1
  Compare To Constant1/1 -> y_h_max_oper/1
  y_h/1 -> Compare To Constant3/1, Compare To Constant2/1, Compare To Constant1/1, Compare To Constant/1
  Compare To Constant3/1 -> y_h_max_emer/1

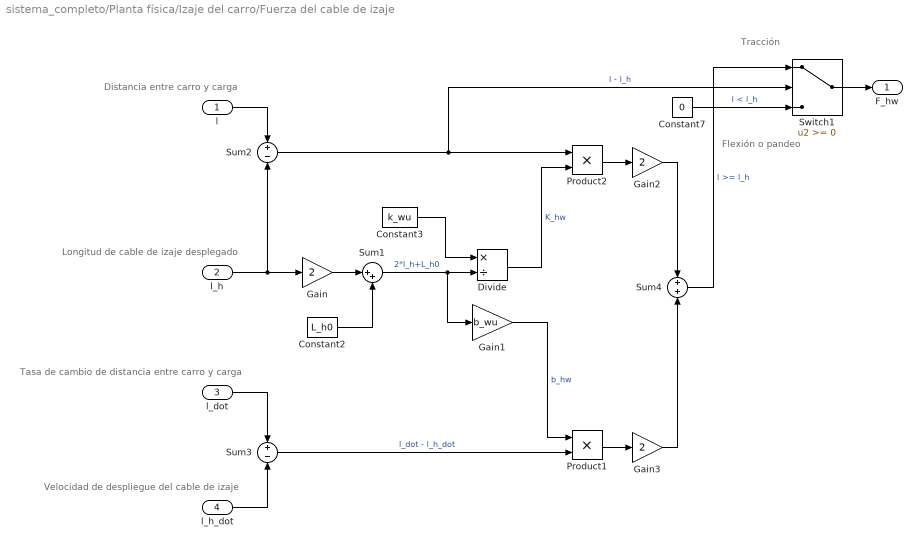
== system sistema_completo/Planta física/Izaje del carro/Fuerza del cable de izaje ==
  note: Flexión o pandeo
  note: Tracción
  note: Distancia entre carro y carga
  note: Tasa de cambio de distancia entre carro y carga
  note: Longitud de cable de izaje desplegado
  note: Velocidad de despliegue del cable de izaje
  l : Inport
  l_h : Inport  Port=2
  l_dot : Inport  Port=3
  l_h_dot : Inport  Port=4
  Constant2 : Constant  Value=L_h0
  Constant3 : Constant  Value=k_wu
  Constant7 : Constant  Value=0
  Divide : Product  Inputs=*/
  Gain : Gain  Gain=2
  Gain1 : Gain  Gain=b_wu
  Gain2 : Gain  Gain=2
  Gain3 : Gain  Gain=2
  Product1 : Product
  Product2 : Product
  Sum1 : Sum  Inputs=|++
  Sum2 : Sum  Inputs=+-
  Sum3 : Sum  Inputs=+-
  Sum4 : Sum
  Switch1 : Switch
  F_hw : Outport
  wires:
  l_dot/1 -> Sum3/1
  Constant2/1 -> Sum1/2
  Sum1/1 -> Gain1/1, Divide/2  "2*l_h+L_h0"
  l/1 -> Sum2/1
  Product1/1 -> Gain3/1
  Sum3/1 -> Product1/2  "l_dot - l_h_dot"
  l_h_dot/1 -> Sum3/2
  l_h/1 -> Gain/1, Sum2/2
  Divide/1 -> Product2/2  "K_hw"
  Sum2/1 -> Switch1/2, Product2/1  "l - l_h"
  Constant3/1 -> Divide/1
  Gain1/1 -> Product1/1  "b_hw"
  Product2/1 -> Gain2/1
  Switch1/1 -> F_hw/1
  Sum4/1 -> Switch1/1  "l >= l_h"
  Constant7/1 -> Switch1/3  "l < l_h"
  Gain/1 -> Sum1/1
  Gain2/1 -> Sum4/1
  Gain3/1 -> Sum4/2

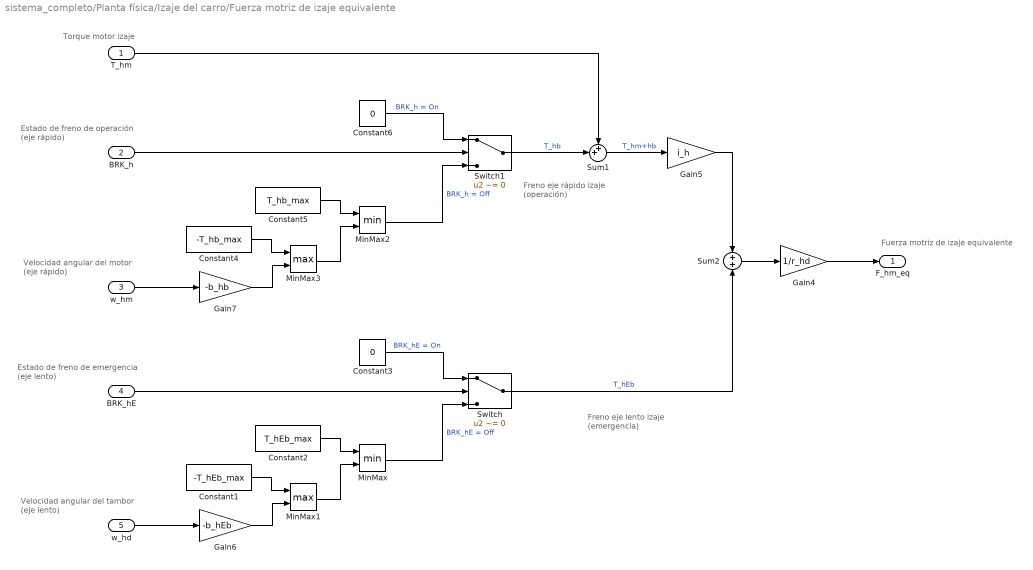
== system sistema_completo/Planta física/Izaje del carro/Fuerza motriz de izaje equivalente ==
  note: Fuerza motriz de izaje equivalente
  note: Torque motor izaje
  note: Freno eje lento izaje
      | (emergencia)
  note: Freno eje rápido izaje
      | (operación)
  note: Estado de freno de operación
      | (eje rápido)
  note: Estado de freno de emergencia
      | (eje lento)
  note: Velocidad angular del tambor
      | (eje lento)
  note: Velocidad angular del motor
      | (eje rápido)
  T_hm : Inport
  BRK_h : Inport  Port=2  OutDataTypeStr=boolean
  w_hm : Inport  Port=3
  BRK_hE : Inport  Port=4  OutDataTypeStr=boolean
  w_hd : Inport  Port=5
  Constant1 : Constant  Value=-T_hEb_max
  Constant2 : Constant  Value=T_hEb_max
  Constant3 : Constant  Value=0
  Constant4 : Constant  Value=-T_hb_max
  Constant5 : Constant  Value=T_hb_max
  Constant6 : Constant  Value=0
  Gain4 : Gain  Gain=1/r_hd
  Gain5 : Gain  Gain=i_h
  Gain6 : Gain  Gain=-b_hEb
  Gain7 : Gain  Gain=-b_hb
  MinMax : MinMax  Inputs=2
  MinMax1 : MinMax  Function=max  Inputs=2
  MinMax2 : MinMax  Inputs=2
  MinMax3 : MinMax  Function=max  Inputs=2
  Sum1 : Sum  Inputs=++|
  Sum2 : Sum  Inputs=2
  Switch : Switch  Criteria=u2 ~= 0
  Switch1 : Switch  Criteria=u2 ~= 0
  F_hm_eq : Outport
  wires:
  MinMax3/1 -> MinMax2/2
  MinMax1/1 -> MinMax/2
  Constant1/1 -> MinMax1/1
  MinMax2/1 -> Switch1/3  "BRK_h = Off"
  Gain5/1 -> Sum2/1
  Constant4/1 -> MinMax3/1
  T_hm/1 -> Sum1/1
  w_hm/1 -> Gain7/1
  Constant5/1 -> MinMax2/1
  w_hd/1 -> Gain6/1
  Gain7/1 -> MinMax3/2
  BRK_h/1 -> Switch1/2
  Constant6/1 -> Switch1/1  "BRK_h = On"
  MinMax/1 -> Switch/3  "BRK_hE = Off"
  Sum1/1 -> Gain5/1  "T_hm+hb"
  Switch1/1 -> Sum1/2  "T_hb"
  Constant3/1 -> Switch/1  "BRK_hE = On"
  BRK_hE/1 -> Switch/2
  Constant2/1 -> MinMax/1
  Gain6/1 -> MinMax1/2
  Gain4/1 -> F_hm_eq/1
  Sum2/1 -> Gain4/1
  Switch/1 -> Sum2/2  "T_hEb"

== system sistema_completo/Planta física/Izaje del carro/Modulador de torque en accionamiento de izaje ==
  note: Modelo de torque idealizado equivalente,
      | modelo simplificado de primer orden LTI en tiempo continuo
  note: Consigna de torque de motor de izaje
  note: Velocidad del motor de izaje
  note: Torque de motor de izaje
  T_hm* : Inport
  w_hm : Inport  Port=2
  Gain1 : Gain  Gain=1/tau_hm
  Gain3 : Gain  Gain=-1
  Integrator2 : Integrator
  Limitador de torque máximo en tiempo discretizado : Subsystem
  Reducción cuadrática de torque máximo (field weakening) : Subsystem
  Sum : Sum  Inputs=|++
  T_hm : Outport
  wires:
  Integrator2/1 -> T_hm/1, Gain3/1  "T_hm"
  Gain3/1 -> Sum/2
  Gain1/1 -> Integrator2/1  "T_hm_dot"
  Sum/1 -> Gain1/1
  Limitador de torque máximo en tiempo discretizado/1(T_hm_lim*) -> Sum/1  "T_hm_lim*"
  Reducción cuadrática de torque máximo (field weakening)/1(T_hm_max) -> Limitador de torque máximo en tiempo discretizado/1(T_hm_max)  "T_hm_max"
  T_hm*/1 -> Limitador de torque máximo en tiempo discretizado/2(T_hm*)  "T_hm*"
  w_hm/1 -> Reducción cuadrática de torque máximo (field weakening)/1(w_hm)  "w_hm"
